simulink model "sampleModel1912_2_sub_sub"  (R2023a)
settings: Solver=VariableStepAuto  StartTime=0.0  StopTime=10.0  RelTol=1e-3
libraries: simulink x5, hdlsllib x3
settings Model: Creator=user1  LastModifiedBy=user1

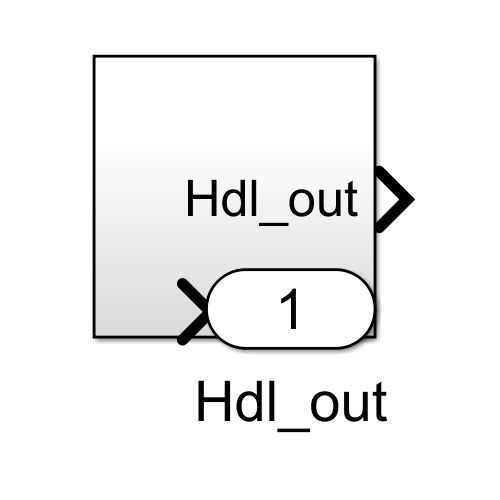
[thumbnail: Simulink's stored preview of the top-level diagram]
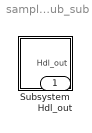
== system sampleModel1912_2_sub_sub ==
  Subsystem : Subsystem
  Hdl_out : Outport  OutDataTypeStr=uint8

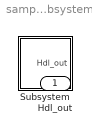
== system sampleModel1912_2_sub_sub/Subsystem ==
  Subsystem : Subsystem
  Hdl_out : Outport  OutDataTypeStr=uint8

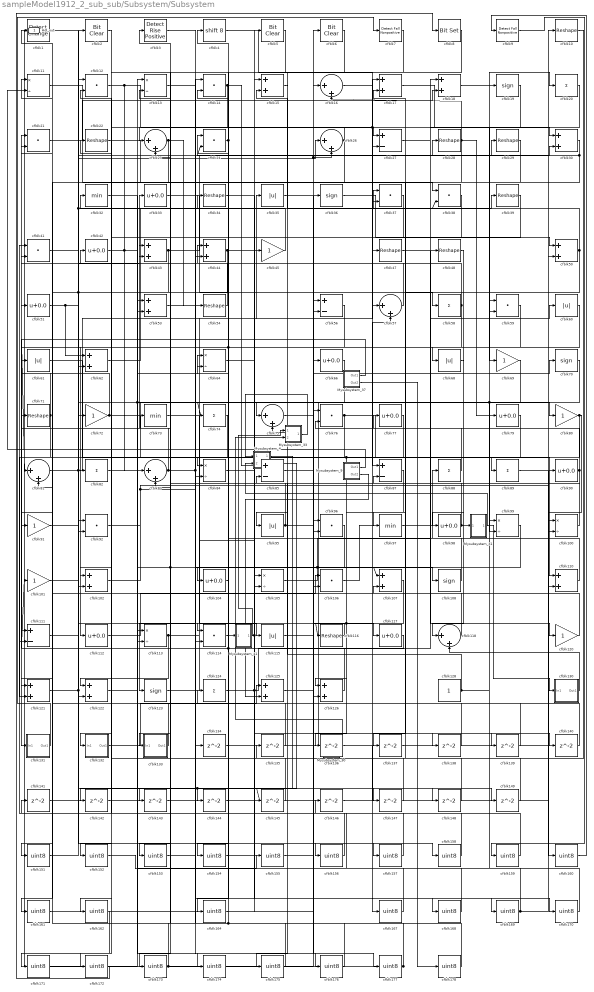
== system sampleModel1912_2_sub_sub/Subsystem/Subsystem ==
  Mysubsystem_30 : Subsystem  TreatAsAtomicUnit=on  RTWFcnName=Mysubsystem_30
      settings: RTWFcnNameOpts=User specified  RTWFileNameOpts=Use function name
  Mysubsystem_31 : Subsystem  TreatAsAtomicUnit=on  RTWFcnName=Mysubsystem_31
      settings: RTWFcnNameOpts=User specified  RTWFileNameOpts=Use function name
  Mysubsystem_33 : Subsystem  TreatAsAtomicUnit=on  RTWFcnName=Mysubsystem_33
      settings: RTWFcnNameOpts=User specified  RTWFileNameOpts=Use function name
  Mysubsystem_37 : Subsystem  TreatAsAtomicUnit=on  RTWFcnName=Mysubsystem_37
      settings: RTWFcnNameOpts=User specified  RTWFileNameOpts=Use function name
  Mysubsystem_4 : Subsystem  TreatAsAtomicUnit=on  RTWFcnName=Mysubsystem_4
      settings: RTWFcnNameOpts=User specified  RTWFileNameOpts=Use function name
  Mysubsystem_41 : Subsystem  TreatAsAtomicUnit=on  RTWFcnName=Mysubsystem_41
      settings: RTWFcnNameOpts=User specified  RTWFileNameOpts=Use function name
  Mysubsystem_9 : Subsystem  TreatAsAtomicUnit=on  RTWFcnName=Mysubsystem_9
      settings: RTWFcnNameOpts=User specified  RTWFileNameOpts=Use function name
  cfblk1 : simulink/Logic and Bit Operations/Detect Change  vinit=0  OutDataTypeStr=uint8
      settings: LibrarySourceBlock=|
      | hdlsllib/Logic and Bit
      | Operations/Detect
      | Change
  cfblk{10,22,28..29,34,39,47..48,54,71,116} (11 alike) : Reshape
  cfblk{11,13,64,84,99..100,105,113} (8 alike) : Product  Inputs=*/  OutDataTypeStr=uint8  RndMeth=Zero  SaturateOnIntegerOverflow=on
  cfblk{45,69,72,80,91,101,120} (7 alike) : Gain  OutDataTypeStr=uint8
  cfblk{15,17..18,30,43..44,50,53,62,102,107,110,121..122,125..126} (16 alike) : Sum  OutDataTypeStr=uint8
  cfblk{33,42,51,66,77,79,90,98,104,112,117} (11 alike) : Bias  Bias=0.0  SaturateOnIntegerOverflow=off
  cfblk{12,14,21,24,37..38,41,59,76,92,96,106,114} (13 alike) : DotProduct  OutDataTypeStr=uint8
  cfblk{19,36,70,108,123} (5 alike) : Signum
  cfblk{27,56,85,87,111} (5 alike) : Sum  Inputs=+-  OutDataTypeStr=uint8
  cfblk{35,60..61,68,95,115} (6 alike) : Abs  OutDataTypeStr=uint8  SaturateOnIntegerOverflow=off
  cfblk{16,23,26,57,75,81,83,118} (8 alike) : Sum  Inputs=|++  OutDataTypeStr=uint8
  cfblk{20,58,74,82,88..89,124} (7 alike) : Sum  Inputs=+  OutDataTypeStr=uint8
  cfblk128 : Constant  OutDataTypeStr=uint8  SampleTime=-1
  cfblk130 : Subsystem
      settings: LibrarySourceBlock=|
      | hdlsllib/Ports &
      | Subsystems/Subsystem
  cfblk131 : Subsystem
      settings: LibrarySourceBlock=|
      | hdlsllib/Ports &
      | Subsystems/Subsystem
  cfblk132 : Subsystem
      settings: LibrarySourceBlock=|
      | hdlsllib/Ports &
      | Subsystems/Subsystem
  cfblk133 : Subsystem
      settings: LibrarySourceBlock=|
      | hdlsllib/Ports &
      | Subsystems/Subsystem
  cfblk{134..149} (16 alike) : Delay  SampleTime=1
  cfblk{151..162,164,167..178} (25 alike) : DataTypeConversion  OutDataTypeStr=uint8  SaturateOnIntegerOverflow=off  RndMeth=Floor
  cfblk2 : simulink/Logic and Bit Operations/Bit Clear  iBit=0
      settings: LibrarySourceBlock=|
      | hdlsllib/Logic and Bit
      | Operations/Bit Clear
  cfblk3 : hdlsllib/Logic and Bit Operations/Detect Rise Positive  vinit=0  OutDataTypeStr=uint8
  cfblk32 : MinMax  OutDataTypeStr=uint8
  cfblk4 : ArithShift  BitShiftNumber=8
  cfblk5 : simulink/Logic and Bit Operations/Bit Clear  iBit=0
      settings: LibrarySourceBlock=|
      | hdlsllib/Logic and Bit
      | Operations/Bit Clear
  cfblk6 : simulink/Logic and Bit Operations/Bit Clear  iBit=0
      settings: LibrarySourceBlock=|
      | hdlsllib/Logic and Bit
      | Operations/Bit Clear
  cfblk7 : hdlsllib/Logic and Bit Operations/Detect Fall Nonpositive  vinit=0  OutDataTypeStr=uint8
  cfblk73 : MinMax  OutDataTypeStr=uint8
  cfblk8 : simulink/Logic and Bit Operations/Bit Set  iBit=0
      settings: LibrarySourceBlock=|
      | hdlsllib/Logic and Bit
      | Operations/Bit Set
  cfblk9 : hdlsllib/Logic and Bit Operations/Detect Fall Nonpositive  vinit=0  OutDataTypeStr=uint8
  cfblk97 : MinMax  OutDataTypeStr=uint8
  Hdl_out : Outport  OutDataTypeStr=uint8
  wires:
  Mysubsystem_41/1(Out1) -> Mysubsystem_33/1(In1)
  Mysubsystem_37/2(Out2) -> cfblk178/1
  Mysubsystem_37/1(Out1) -> cfblk131/1(In1)
  Mysubsystem_33/1(Out1) -> Mysubsystem_4/1(In1)
  Mysubsystem_30/1(Out1) -> Mysubsystem_33/2(In2)
  Mysubsystem_31/1(Out1) -> Mysubsystem_4/2(In2)
  cfblk106/1 -> Mysubsystem_31/1(In1)
  cfblk66/1 -> Mysubsystem_30/1(In1)
  Mysubsystem_9/2(Out2) -> cfblk125/2
  Mysubsystem_9/1(Out1) -> cfblk11/2
  Mysubsystem_4/2(Out2) -> cfblk143/1
  Mysubsystem_4/1(Out1) -> cfblk142/1
  cfblk178/1 -> cfblk13/2
  cfblk177/1 -> cfblk13/1, Hdl_out/1
  cfblk176/1 -> cfblk14/1
  cfblk13/1 -> cfblk176/1
  cfblk175/1 -> cfblk113/1, cfblk124/1
  cfblk174/1 -> cfblk6/1
  cfblk122/1 -> cfblk174/1
  cfblk173/1 -> cfblk141/1, cfblk106/2
  cfblk172/1 -> cfblk8/1
  cfblk171/1 -> cfblk53/2
  cfblk162/1 -> cfblk171/1
  cfblk170/1 -> cfblk53/1
  cfblk136/1 -> cfblk170/1
  cfblk169/1 -> cfblk100/2, cfblk59/1
  cfblk168/1 -> cfblk146/1
  cfblk34/1 -> cfblk168/1
  cfblk167/1 -> cfblk76/1
  cfblk146/1 -> cfblk167/1
  cfblk164/1 -> cfblk66/1
  cfblk77/1 -> cfblk164/1
  cfblk5/1 -> cfblk162/1
  cfblk161/1 -> cfblk5/1
  cfblk160/1 -> cfblk9/1
  cfblk89/1 -> cfblk160/1
  cfblk159/1 -> cfblk42/1
  cfblk9/1 -> cfblk159/1
  cfblk158/1 -> cfblk41/2
  cfblk157/1 -> cfblk41/1
  cfblk3/1 -> cfblk157/1
  cfblk156/1 -> cfblk14/2
  cfblk41/1 -> cfblk156/1
  cfblk155/1 -> cfblk96/2
  cfblk152/1 -> cfblk155/1
  cfblk154/1 -> cfblk96/1
  cfblk153/1 -> cfblk134/1
  cfblk96/1 -> cfblk153/1
  cfblk2/1 -> cfblk152/1
  cfblk151/1 -> cfblk2/1
  cfblk149/1 -> cfblk105/1
  cfblk148/1 -> cfblk107/2
  cfblk147/1 -> cfblk15/1
  cfblk145/1 -> cfblk12/2
  cfblk144/1 -> cfblk56/1
  cfblk143/1 -> cfblk59/2
  cfblk142/1 -> cfblk57/2
  cfblk141/1 -> cfblk50/2
  cfblk140/1 -> cfblk99/1
  cfblk35/1 -> cfblk140/1
  cfblk139/1 -> cfblk1/1
  cfblk64/1 -> cfblk139/1
  cfblk138/1 -> cfblk83/2
  cfblk84/1 -> cfblk138/1
  cfblk137/1 -> cfblk17/2
  cfblk87/1 -> cfblk136/1
  cfblk135/1 -> cfblk92/1
  cfblk10/1 -> cfblk135/1
  cfblk134/1 -> cfblk110/2
  cfblk97/1 -> cfblk60/1
  cfblk108/1 -> cfblk24/1
  cfblk28/1 -> cfblk16/2, cfblk75/2, cfblk79/1
  cfblk133/1(Out1) -> cfblk111/1
  cfblk39/1 -> cfblk104/1
  cfblk6/1 -> cfblk175/1
  cfblk82/1 -> cfblk64/2
  cfblk24/1 -> Mysubsystem_41/1(In1), cfblk4/1
  cfblk88/1 -> cfblk76/2
  cfblk20/1 -> cfblk84/2
  cfblk91/1 -> cfblk114/2
  cfblk56/1 -> cfblk132/1(In1)
  cfblk90/1 -> cfblk87/2, cfblk77/1
  cfblk104/1 -> cfblk64/1
  cfblk29/1 -> cfblk91/1
  cfblk37/1 -> cfblk82/1
  cfblk80/1 -> cfblk100/1, cfblk126/2
  cfblk50/1 -> cfblk15/2, cfblk97/1
  cfblk120/1 -> cfblk3/1
  cfblk1/1 -> cfblk72/1
  cfblk92/1 -> cfblk10/1, cfblk44/2
  cfblk68/1 -> cfblk98/1
  cfblk57/1 -> cfblk22/1
  cfblk44/1 -> cfblk62/2, cfblk161/1, cfblk158/1
  cfblk21/1 -> cfblk18/2
  cfblk32/1 -> cfblk74/1, cfblk149/1
  cfblk18/1 -> cfblk20/1
  cfblk51/1 -> cfblk43/2, cfblk62/1
  cfblk115/1 -> cfblk56/2
  cfblk111/1 -> cfblk12/1
  cfblk30/1 -> cfblk24/2, cfblk137/1
  cfblk76/1 -> cfblk89/1, cfblk81/2
  cfblk81/1 -> cfblk17/1, cfblk26/1
  cfblk75/1 -> cfblk70/1
  cfblk121/1 -> cfblk29/1, cfblk38/2, cfblk148/1
  cfblk4/1 -> cfblk57/1
  cfblk85/1 -> cfblk117/1
  cfblk99/1 -> cfblk133/1(In1), cfblk113/2
  cfblk74/1 -> cfblk121/2
  cfblk95/1 -> cfblk43/1, cfblk177/1
  cfblk26/1 -> cfblk23/1, cfblk102/2
  cfblk27/1 -> cfblk30/1
  cfblk11/1 -> cfblk38/1
  cfblk79/1 -> cfblk126/1, cfblk116/1, cfblk121/1
  cfblk54/1 -> cfblk11/1
  cfblk126/1 -> cfblk101/1, cfblk34/1
  cfblk7/1 -> cfblk84/1
  cfblk71/1 -> cfblk51/1, cfblk111/2
  cfblk61/1 -> cfblk90/1
  cfblk47/1 -> cfblk120/1
  cfblk69/1 -> cfblk92/2
  cfblk107/1 -> cfblk123/1
  cfblk116/1 -> cfblk114/1
  cfblk14/1 -> cfblk122/1, cfblk85/1
  cfblk132/1(Out1) -> cfblk125/1
  cfblk123/1 -> cfblk45/1
  cfblk60/1 -> cfblk68/1
  cfblk105/1 -> cfblk18/1, cfblk107/1
  cfblk58/1 -> cfblk81/1, cfblk154/1, cfblk44/1
  cfblk33/1 -> cfblk58/1
  cfblk130/1(Out1) -> cfblk118/2
  cfblk70/1 -> cfblk99/2, cfblk105/2
  cfblk131/1(Out1) -> cfblk7/1
  cfblk15/1 -> cfblk95/1
  cfblk48/1 -> cfblk118/1
  cfblk38/1 -> cfblk102/1
  cfblk22/1 -> cfblk47/1
  cfblk16/1 -> cfblk87/1
  cfblk118/1 -> cfblk21/2
  cfblk8/1 -> cfblk173/1
  cfblk100/1 -> cfblk37/1
  cfblk17/1 -> cfblk69/1
  cfblk112/1 -> cfblk36/1
  cfblk45/1 -> cfblk32/1
  cfblk19/1 -> cfblk27/2, cfblk23/2
  cfblk124/1 -> cfblk48/1, cfblk37/2
  cfblk125/1 -> cfblk16/1, cfblk26/2
  cfblk43/1 -> cfblk28/1, cfblk122/2
  cfblk114/1 -> cfblk106/1, cfblk147/1
  cfblk53/1 -> cfblk169/1
  cfblk59/1 -> cfblk112/1
  cfblk12/1 -> cfblk27/1, cfblk73/1
  cfblk110/1 -> cfblk88/1
  cfblk128/1 -> cfblk19/1, cfblk85/2
  cfblk62/1 -> cfblk39/1
  cfblk101/1 -> cfblk144/1, cfblk145/1
  cfblk36/1 -> cfblk50/1
  cfblk113/1 -> cfblk35/1, cfblk172/1
  cfblk83/1 -> cfblk30/2, cfblk108/1, cfblk33/1
  cfblk98/1 -> cfblk130/1(In1), cfblk71/1
  cfblk23/1 -> cfblk54/1, cfblk151/1
  cfblk72/1 -> cfblk110/1, cfblk61/1
  cfblk117/1 -> cfblk21/1
  cfblk102/1 -> cfblk80/1
  cfblk73/1 -> cfblk115/1
  cfblk42/1 -> cfblk83/1, cfblk75/1

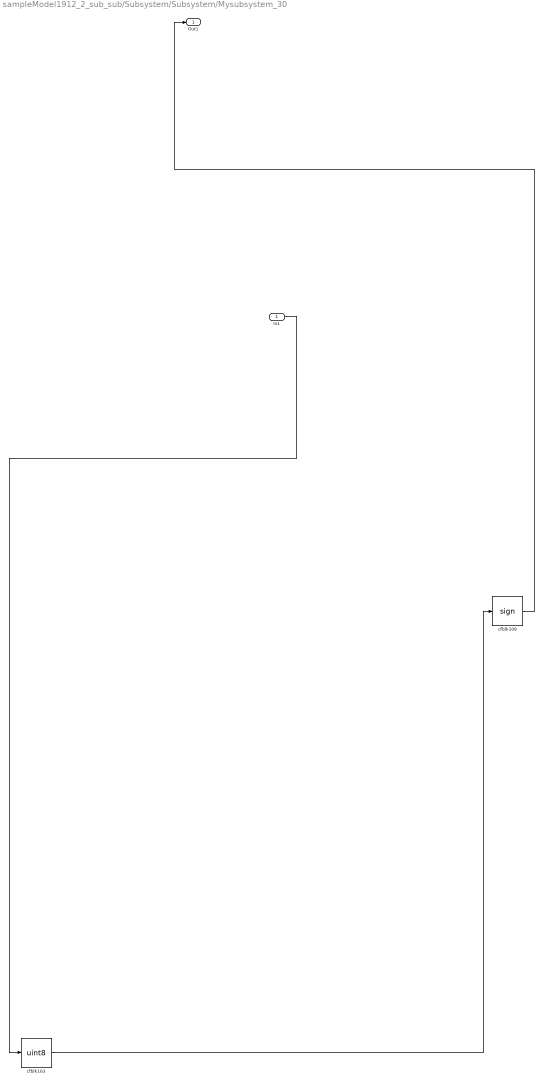
== system sampleModel1912_2_sub_sub/Subsystem/Subsystem/Mysubsystem_30 ==
  In1 : Inport
  cfblk109 : Signum
  cfblk163 : DataTypeConversion  OutDataTypeStr=uint8  SaturateOnIntegerOverflow=off  RndMeth=Floor
  Out1 : Outport
  wires:
  cfblk163/1 -> cfblk109/1
  cfblk109/1 -> Out1/1
  In1/1 -> cfblk163/1

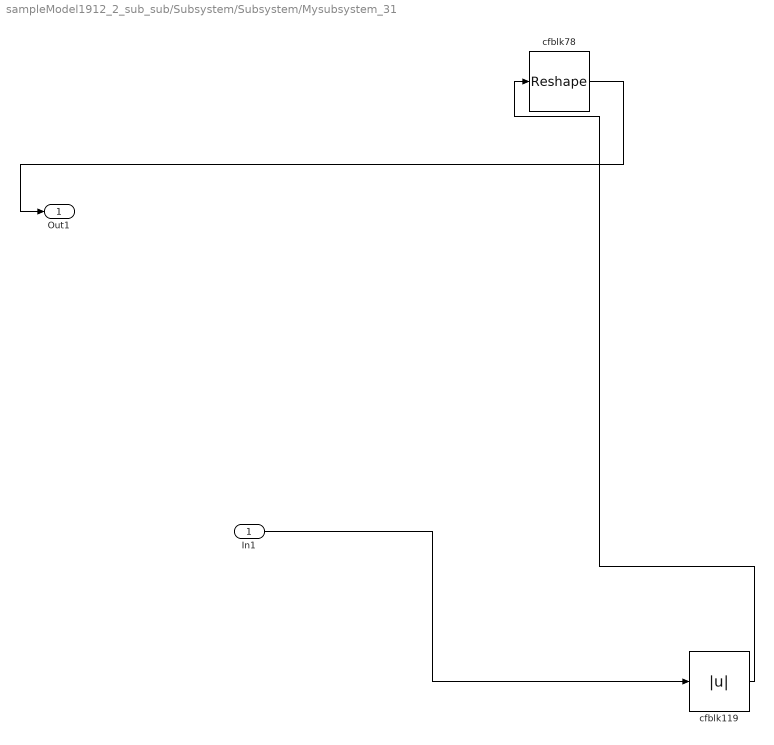
== system sampleModel1912_2_sub_sub/Subsystem/Subsystem/Mysubsystem_31 ==
  In1 : Inport
  cfblk119 : Abs  SaturateOnIntegerOverflow=off
  cfblk78 : Reshape
  Out1 : Outport
  wires:
  cfblk119/1 -> cfblk78/1
  In1/1 -> cfblk119/1
  cfblk78/1 -> Out1/1

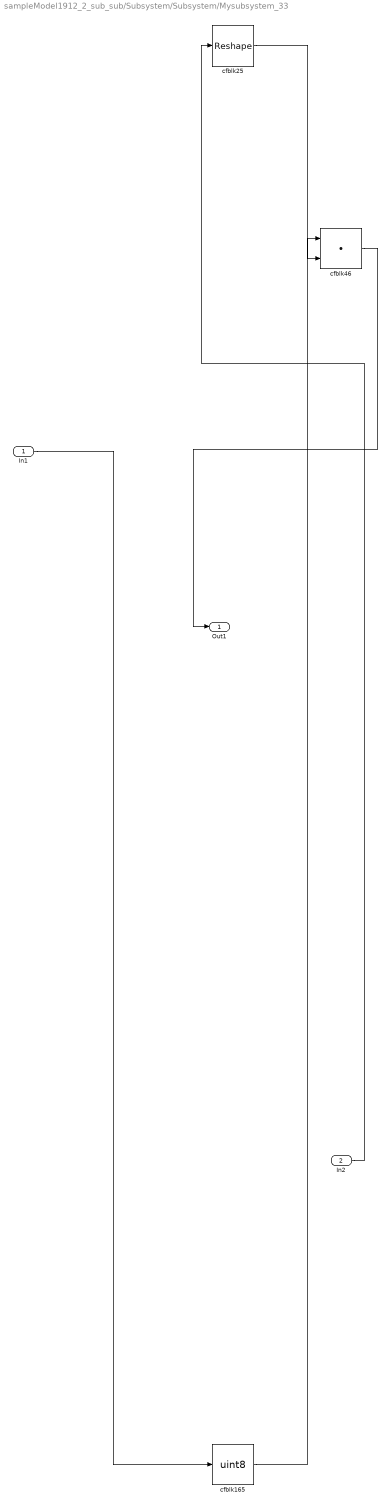
== system sampleModel1912_2_sub_sub/Subsystem/Subsystem/Mysubsystem_33 ==
  In1 : Inport
  In2 : Inport  Port=2
  cfblk165 : DataTypeConversion  OutDataTypeStr=uint8  SaturateOnIntegerOverflow=off  RndMeth=Floor
  cfblk25 : Reshape
  cfblk46 : DotProduct  OutDataTypeStr=Inherit: Inherit via internal rule
  Out1 : Outport
  wires:
  cfblk25/1 -> cfblk46/2
  In1/1 -> cfblk165/1
  cfblk165/1 -> cfblk46/1
  cfblk46/1 -> Out1/1
  In2/1 -> cfblk25/1

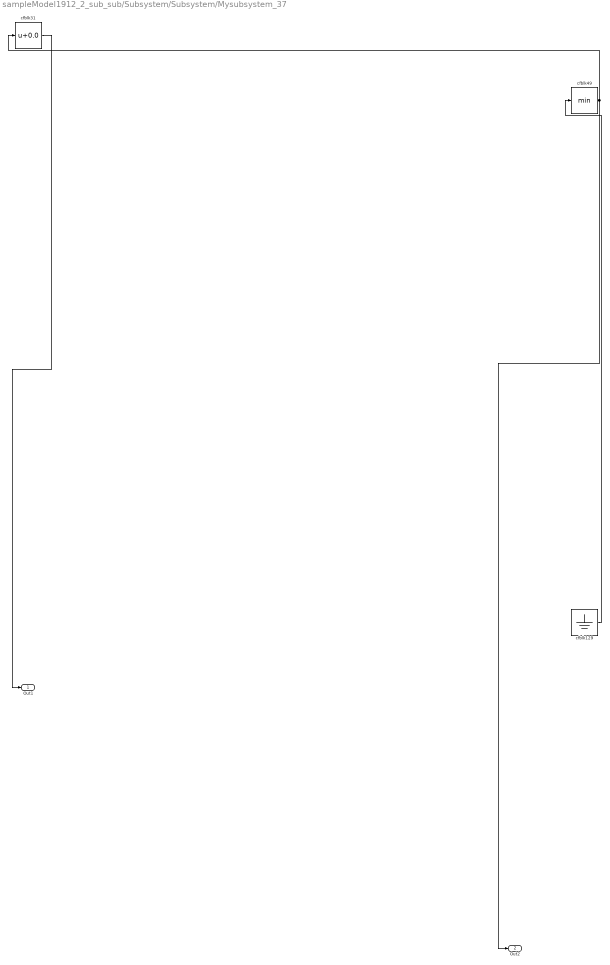
== system sampleModel1912_2_sub_sub/Subsystem/Subsystem/Mysubsystem_37 ==
  cfblk129 : Ground
  cfblk31 : Bias  Bias=0.0  SaturateOnIntegerOverflow=off
  cfblk49 : MinMax
  Out1 : Outport
  Out2 : Outport  Port=2
  wires:
  cfblk129/1 -> cfblk49/1
  cfblk49/1 -> Out2/1, cfblk31/1
  cfblk31/1 -> Out1/1

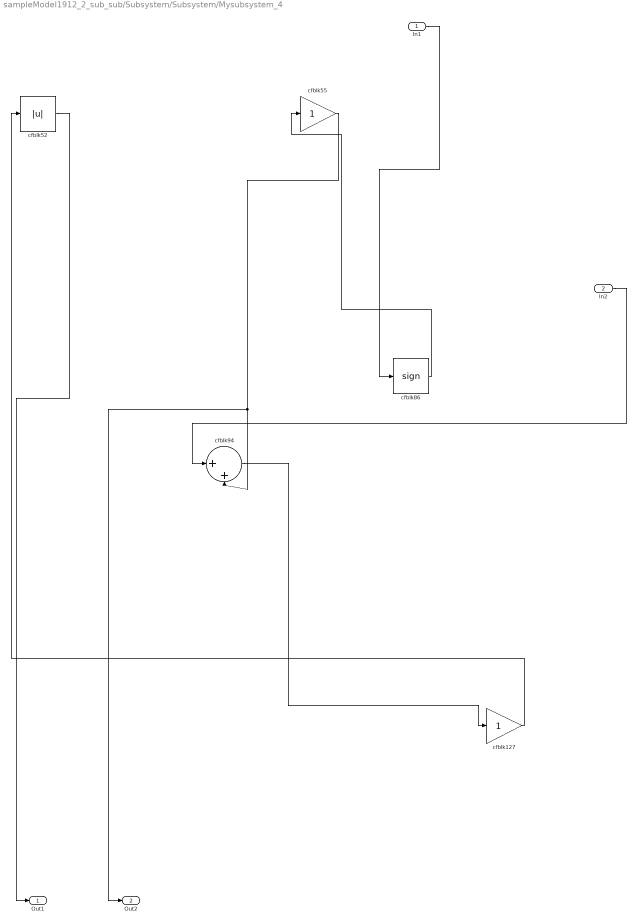
== system sampleModel1912_2_sub_sub/Subsystem/Subsystem/Mysubsystem_4 ==
  In1 : Inport
  In2 : Inport  Port=2
  cfblk127 : Gain
  cfblk52 : Abs  SaturateOnIntegerOverflow=off
  cfblk55 : Gain
  cfblk86 : Signum
  cfblk94 : Sum  Inputs=|++
  Out1 : Outport
  Out2 : Outport  Port=2
  wires:
  cfblk86/1 -> cfblk55/1
  cfblk127/1 -> cfblk52/1
  In1/1 -> cfblk86/1
  In2/1 -> cfblk94/1
  cfblk94/1 -> cfblk127/1
  cfblk55/1 -> Out2/1, cfblk94/2
  cfblk52/1 -> Out1/1

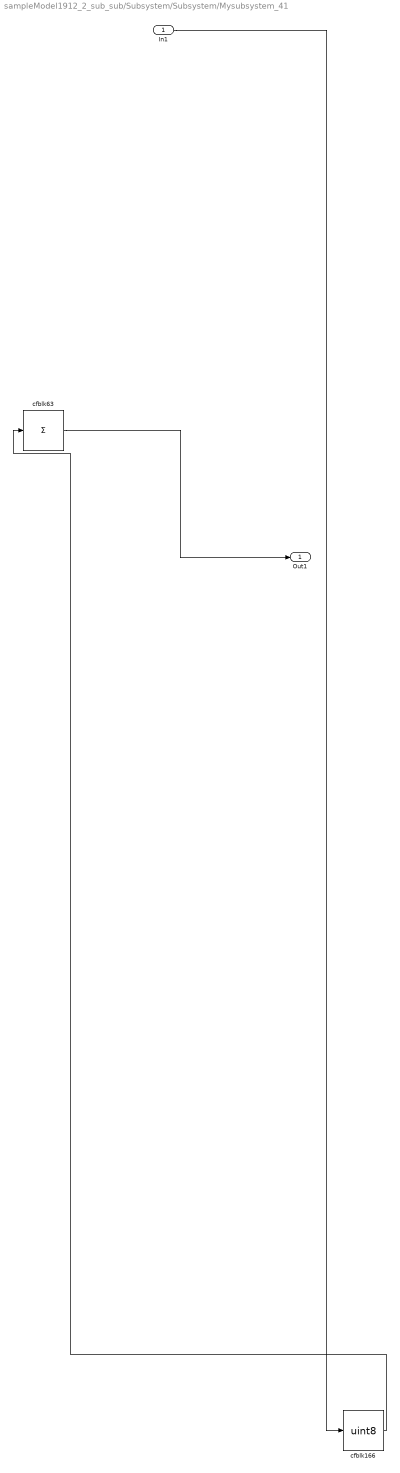
== system sampleModel1912_2_sub_sub/Subsystem/Subsystem/Mysubsystem_41 ==
  In1 : Inport
  cfblk166 : DataTypeConversion  OutDataTypeStr=uint8  SaturateOnIntegerOverflow=off  RndMeth=Floor
  cfblk63 : Sum  Inputs=+
  Out1 : Outport
  wires:
  cfblk63/1 -> Out1/1
  cfblk166/1 -> cfblk63/1
  In1/1 -> cfblk166/1

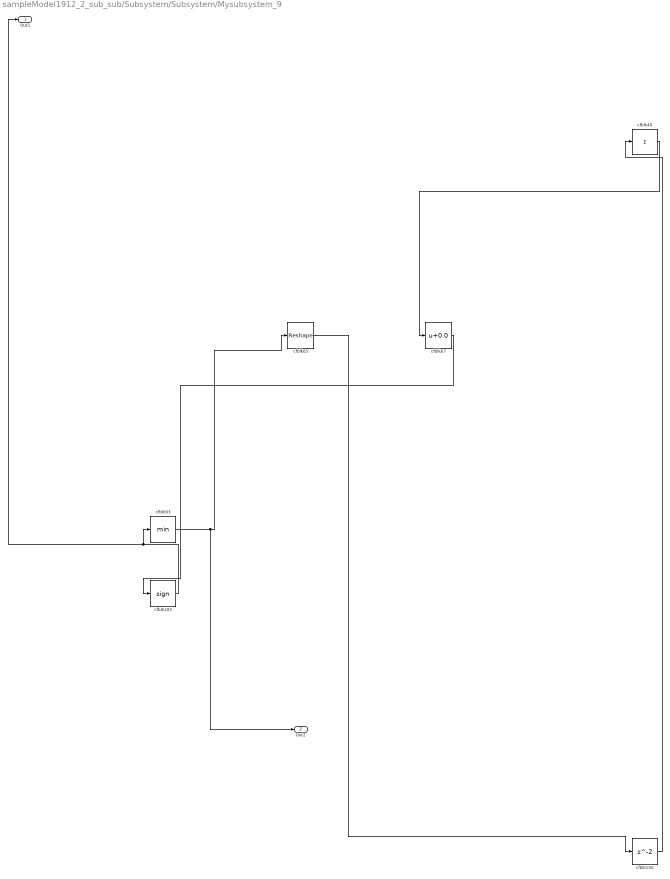
== system sampleModel1912_2_sub_sub/Subsystem/Subsystem/Mysubsystem_9 ==
  cfblk103 : Signum
  cfblk150 : Delay  SampleTime=1
  cfblk40 : Sum  Inputs=+
  cfblk65 : Reshape
  cfblk67 : Bias  Bias=0.0  SaturateOnIntegerOverflow=off
  cfblk93 : MinMax
  Out1 : Outport
  Out2 : Outport  Port=2
  wires:
  cfblk93/1 -> Out2/1, cfblk65/1
  cfblk103/1 -> Out1/1, cfblk93/1
  cfblk40/1 -> cfblk67/1
  cfblk150/1 -> cfblk40/1
  cfblk65/1 -> cfblk150/1
  cfblk67/1 -> cfblk103/1

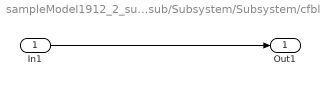
== system sampleModel1912_2_sub_sub/Subsystem/Subsystem/cfblk130 ==
  In1 : Inport
  Out1 : Outport
  wires:
  In1/1 -> Out1/1

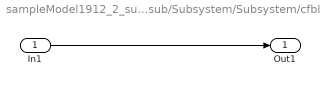
== system sampleModel1912_2_sub_sub/Subsystem/Subsystem/cfblk131 ==
  In1 : Inport
  Out1 : Outport
  wires:
  In1/1 -> Out1/1

== system sampleModel1912_2_sub_sub/Subsystem/Subsystem/cfblk132 ==
  In1 : Inport
  Out1 : Outport
  wires:
  In1/1 -> Out1/1

== system sampleModel1912_2_sub_sub/Subsystem/Subsystem/cfblk133 ==
  In1 : Inport
  Out1 : Outport
  wires:
  In1/1 -> Out1/1
